simulink model "three_Phase_inverter_Mathematcial_Model"  (R2021a)
settings: Solver=VariableStepAuto  StartTime=0.0  StopTime=.08  RelTol=1e-3
InitFcn:
  | Vdc=200
libraries: spsIGBTDiodeLib x6, spsCurrentMeasurementLib x3, spsSeriesRLCBranchLib x3, spsVoltageMeasurementLib x2, spsDCVoltageSourceLib x1, spsTriangleGeneratorLib x1, spspowerguiLib x1
settings Model: Creator=User  LastModifiedBy=User

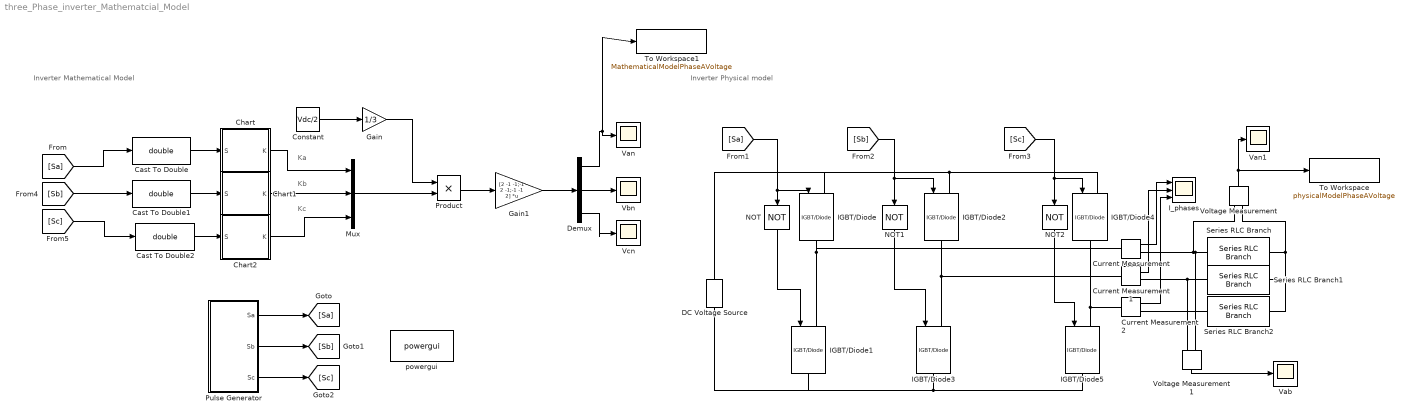
== system three_Phase_inverter_Mathematcial_Model ==
  note: Ka
  note: Inverter Physical model
  note: Inverter Mathematical Model
  note: Kb
  note: Kc
  Cast To Double : DataTypeConversion  OutDataTypeStr=double
  Cast To Double1 : DataTypeConversion  OutDataTypeStr=double
  Cast To Double2 : DataTypeConversion  OutDataTypeStr=double
  Chart : Stateflow chart  TreatAsAtomicUnit=on
  Chart1 : Stateflow chart  TreatAsAtomicUnit=on
  Chart2 : Stateflow chart  TreatAsAtomicUnit=on
  Constant : Constant  Value=Vdc/2
  Current Measurement : spsCurrentMeasurementLib/Current Measurement  PhasorSimulation=off  OutputType=Complex  PSBequivalent=0
  Current Measurement1 : spsCurrentMeasurementLib/Current Measurement  PhasorSimulation=off  OutputType=Complex  PSBequivalent=0
  Current Measurement2 : spsCurrentMeasurementLib/Current Measurement  PhasorSimulation=off  OutputType=Complex  PSBequivalent=0
  DC Voltage Source : spsDCVoltageSourceLib/DC Voltage Source  Amplitude=Vdc  Measurements=None
  Demux : Demux  Outputs=3
  Gain : Gain  Gain=1/3
  Gain1 : Gain  Gain=[2 -1 -1;-1 2 -1;-1 -1 2]  Multiplication=Matrix(K*u)
  IGBT/Diode{,1..5} (6 alike) : spsIGBTDiodeLib/IGBT//Diode  Ron=1e-3  Rs=1e5  Cs=inf  Measurements=off
  I_phases : Scope  NumInputPorts=3
  Mux : Mux  Inputs=3
  NOT : Logic  Operator=NOT  IconShape=distinctive  AllPortsSameDT=off  OutDataTypeStr=boolean
  NOT1 : Logic  Operator=NOT  IconShape=distinctive  AllPortsSameDT=off  OutDataTypeStr=boolean
  NOT2 : Logic  Operator=NOT  IconShape=distinctive  AllPortsSameDT=off  OutDataTypeStr=boolean
  Product : Product
  Pulse Generator : Subsystem
  Series RLC Branch : spsSeriesRLCBranchLib/Series RLC Branch  LConnTagsString=__new0  RConnTagsString=__new0  BranchType=RL  Resistance=10  Inductance=50e-3  SetiL0=off  InitialCurrent=0  Capacitance=1e-6  Setx0=off  InitialVoltage=0  Measurements=None
  Series RLC Branch1 : spsSeriesRLCBranchLib/Series RLC Branch  LConnTagsString=__new0  RConnTagsString=__new0  BranchType=RL  Resistance=10  Inductance=50e-3  SetiL0=off  InitialCurrent=0  Capacitance=1e-6  Setx0=off  InitialVoltage=0  Measurements=None
  Series RLC Branch2 : spsSeriesRLCBranchLib/Series RLC Branch  LConnTagsString=__new0  RConnTagsString=__new0  BranchType=RL  Resistance=10  Inductance=50e-3  SetiL0=off  InitialCurrent=0  Capacitance=1e-6  Setx0=off  InitialVoltage=0  Measurements=None
  To Workspace : ToWorkspace  VariableName=physicalModelPhaseAVoltage  SaveFormat=Timeseries  SampleTime=-1
  To Workspace1 : ToWorkspace  VariableName=MathematicalModelPhaseAVoltage  SaveFormat=Timeseries  SampleTime=-1
  Vab : Scope
  Van : Scope
  Van1 : Scope
  Vbn : Scope
  Vcn : Scope
  Voltage Measurement : spsVoltageMeasurementLib/Voltage Measurement  PhasorSimulation=off  OutputType=Complex  PSBequivalent=0
  Voltage Measurement1 : spsVoltageMeasurementLib/Voltage Measurement  PhasorSimulation=off  OutputType=Complex  PSBequivalent=0
  powergui : spspowerguiLib/powergui  Priority=1  SimulationMode=Continuous  SampleTime=50e-6  frequency=60  Iterations=50  frequencyindice=0  Pbase=100e6  ErrMax=1e-4  UnitsV=kV  UnitsW=MW  buscounter=0  FunctionMessages=off  echomessages=off  EnableUseOfTLC=off  CurrentSourceSwitches=off  DisableSnubberDevices=off  DisableRonSwitches=off  DisableVfSwitches=off  DisplayEquations=off  AutomaticDiscreteSolvers=off  SolverType=Tustin/Backward Euler (TBE)  Interpol=off  ExternalGateDelay=off  methode=off  Ts=100  x0status=blocks  SPID=on  SwTol=0  HookPort=off  NonlinearTolerance=1e-4  nMaxIteration=100  ContinueOnMaxIteration=off  RestoreLinks=warning  ResistiveCurrentMeasurement=off  Frange=[0:2:500]  Ylog=off  Xlog=on  ShowGrid=off  save=off  variable=ZData  structure=0  ZoomFFT=off  StartTime=0.0  cycles=1  DisplayStyle=1  fundamental=60  FreqAxis=off  MaxFrequency=1000  frequencyindicesteady=1  RmsSteady=1  display=off
  wires:
  Chart1/1(K) -> Mux/2
  Chart/1(K) -> Mux/1
  Chart2/1(K) -> Mux/3
  Mux/1 -> Product/2
  Constant/1 -> Gain/1
  Gain/1 -> Product/1
  Product/1 -> Gain1/1
  Gain1/1 -> Demux/1
  Demux/1 -> To Workspace1/1, Van/1
  Demux/2 -> Vbn/1
  Demux/3 -> Vcn/1
  Cast To Double/1 -> Chart/1(S)
  Cast To Double1/1 -> Chart1/1(S)
  Cast To Double2/1 -> Chart2/1(S)
  [Sa] -> Cast To Double/1
  [Sb] -> Cast To Double1/1
  [Sc] -> Cast To Double2/1
  Pulse Generator/1(Sa) -> [Sa]
  Pulse Generator/2(Sb) -> [Sb]
  Pulse Generator/3(Sc) -> [Sc]
  [Sa] -> NOT/1, IGBT/Diode/1
  NOT/1 -> IGBT/Diode1/1
  [Sb] -> IGBT/Diode2/1, NOT1/1
  NOT1/1 -> IGBT/Diode3/1
  NOT2/1 -> IGBT/Diode5/1
  [Sc] -> NOT2/1, IGBT/Diode4/1
  Voltage Measurement/1 -> To Workspace/1, Van1/1
  Current Measurement/1 -> I_phases/1
  Current Measurement1/1 -> I_phases/2
  Current Measurement2/1 -> I_phases/3
  Voltage Measurement1/1 -> Vab/1
  connections:
  IGBT/Diode4/RConn1 -- Current Measurement2/LConn1 -- IGBT/Diode5/LConn1
  IGBT/Diode2/RConn1 -- Current Measurement1/LConn1 -- IGBT/Diode3/LConn1
  IGBT/Diode/RConn1 -- IGBT/Diode1/LConn1 -- Current Measurement/LConn1
  IGBT/Diode4/LConn1 -- IGBT/Diode/LConn1 -- DC Voltage Source/RConn1 -- IGBT/Diode2/LConn1
  IGBT/Diode5/RConn1 -- DC Voltage Source/LConn1 -- IGBT/Diode1/RConn1 -- IGBT/Diode3/RConn1
  Series RLC Branch/RConn1 -- Voltage Measurement/LConn2 -- Series RLC Branch1/RConn1 -- Series RLC Branch2/RConn1
  Series RLC Branch/LConn1 -- Current Measurement/RConn1 -- Voltage Measurement/LConn1 -- Voltage Measurement1/LConn1
  Current Measurement1/RConn1 -- Voltage Measurement1/LConn2 -- Series RLC Branch1/LConn1
  Current Measurement2/RConn1 -- Series RLC Branch2/LConn1

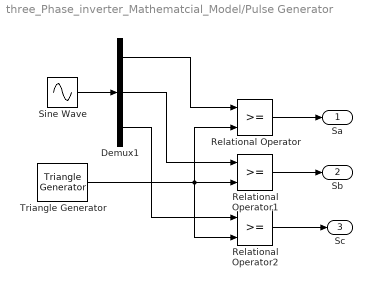
== system three_Phase_inverter_Mathematcial_Model/Pulse Generator ==
  Demux1 : Demux  Outputs=3
  Relational Operator : RelationalOperator  OutDataTypeStr=boolean  RndMeth=Simplest
  Relational Operator1 : RelationalOperator  OutDataTypeStr=boolean  RndMeth=Simplest
  Relational Operator2 : RelationalOperator  OutDataTypeStr=boolean  RndMeth=Simplest
  Sine Wave : Sin  Frequency=2*pi*50  Phase=[0 (2*pi)/3 (-2*pi)/3]  SampleTime=0
  Triangle Generator : spsTriangleGeneratorLib/Triangle Generator  Freq=5e3  Phase=90  Ts=0
  Sa : Outport
  Sb : Outport  Port=2
  Sc : Outport  Port=3
  wires:
  Triangle Generator/1 -> Relational Operator2/2, Relational Operator/2, Relational Operator1/2
  Demux1/1 -> Relational Operator/1
  Demux1/3 -> Relational Operator2/1
  Sine Wave/1 -> Demux1/1
  Demux1/2 -> Relational Operator1/1
  Relational Operator1/1 -> Sb/1
  Relational Operator/1 -> Sa/1
  Relational Operator2/1 -> Sc/1

== stateflow chart three_Phase_inverter_Mathematcial_Model/Chart1 ==
  (default) -> (junction 7) : % determintino of k
  (junction 7) -> (junction 8) [order 1] : [S==0]
  (junction 7) -> (junction 9) [order 2] : {K=1;}
  (junction 8) -> (junction 10) : {
      |       K=-1;
      | }
  (junction 10) -> (junction 9)
  (junction 9) -> (junction 11)
  data: K output; S input

== stateflow chart three_Phase_inverter_Mathematcial_Model/Chart2 ==
  (default) -> (junction 7) : % determintino of k
  (junction 7) -> (junction 8) [order 1] : [S==0]
  (junction 7) -> (junction 9) [order 2] : {K=1;}
  (junction 8) -> (junction 10) : {
      |       K=-1;
      | }
  (junction 10) -> (junction 9)
  (junction 9) -> (junction 11)
  data: K output; S input

== stateflow chart three_Phase_inverter_Mathematcial_Model/Chart ==
  (default) -> (junction 7) : % determintino of k
  (junction 7) -> (junction 8) [order 1] : [S==0]
  (junction 7) -> (junction 9) [order 2] : {K=1;}
  (junction 8) -> (junction 10) : {
      |       K=-1;
      | }
  (junction 10) -> (junction 9)
  (junction 9) -> (junction 11)
  data: K output; S input
